simulink model "S600_stromregelung"  (Simulink 9.2)
settings: Solver=FixedStepDiscrete  StartTime=0.0  StopTime=inf  FixedStep=param.t_sample  RelTol=1e-3
undefined symbols (not defined in the file or in its folder): param
libraries: etherlab_lib x1
settings Model: Creator=schappler  LastModifiedBy=pkr_devpc  SimulationMode=external  ExtModeTrigDuration=10000  ExtModeArchiveMode=auto  ExtModeArchiveFileName=measurement_data  ExtModeArchiveDirName=/home/pkr_devpc/Schreibtisch/Git/3rrr_pkm/Versuchsstand/result  ExtModeLogAll=off
settings SolverCC: MinimalZcImpactIntegration=on
settings DataIOCC: LimitDataPoints=off  SaveFormat=Dataset  SignalLoggingSaveFormat=Dataset  SaveOutput=off  SignalLogging=off  SaveTime=off
settings OptimizationCC: BufferReuse=off  GlobalBufferReuse=off  ExpressionFolding=off  LocalBlockOutputs=off  LifeSpan=auto  OptimizeDataStoreBuffers=off  BusAssignmentInplaceUpdate=off
settings DebuggingCC: ReadBeforeWriteMsg=DisableAll  WriteAfterWriteMsg=DisableAll  WriteAfterReadMsg=DisableAll  UnderspecifiedInitializationDetection=Simplified  MergeDetectMultiDrivingBlocksExec=error  MultiTaskDSMMsg=none  FcnCallInpInsideContextMsg=error  StateNameClashWarn=none  SFUnexpectedBacktrackingDiag=error  SFNoUnconditionalDefaultTransitionDiag=error  SFExecutionAtInitializationDiag=warning
settings HardwareCC: ProdBitPerPointer=64  ProdBitPerSizeT=64  ProdBitPerPtrDiffT=64  ProdLargestAtomicFloat=Float  ProdIntDivRoundTo=Zero  ProdEndianess=LittleEndian  ProdWordSize=64  ProdHWDeviceType=Intel->x86-64 (Windows64)
settings ModelReferenceCC: UpdateModelReferenceTargets=IfOutOfDate  PropagateSignalLabelsOutOfModel=on
settings SFSimCC: SFSimEcho=off  SimUseLocalCustomCode=on
settings RTWCC: SystemTargetFile=etherlab.tlc  TemplateMakefile=etherlab_hrt.tmf  Description=EtherLab PREEMT_RT Real-Time Target  GenerateReport=on  RTWUseLocalCustomCode=on  LaunchReport=on
settings CodeAppCC: StateflowObjectComments=off
settings STFCustomTargetCC: TargetLangStandard=C99 (ISO)  SystemTargetFile=etherlab.tlc
settings GRTTargetCC: TargetLangStandard=C99 (ISO)  ParMdlRefBuildCompliant=off  CompOptLevelCompliant=off  ConcurrentExecutionCompliant=off  GeneratePreprocessorConditionals=Use local settings  MatFileLogging=off  CPPClassGenCompliant=off  UseToolchainInfoCompliant=off  ExtMode=on  ExtModeStaticAlloc=on  ExtModeStaticAllocSize=2000000000  ExtModeMexArgs='10.144.130.139' 0 17725  RTWCAPISignals=on  RTWCAPIParams=on
settings CustomProperty: DataType=int32  Value=2
settings ConfigComp: CovMetricSettings=dwe  CovHtmlReporting=off  CovSaveCumulativeToWorkspaceVar=off  CovSaveSingleToWorkspaceVar=off  CovExternalEMLEnable=on

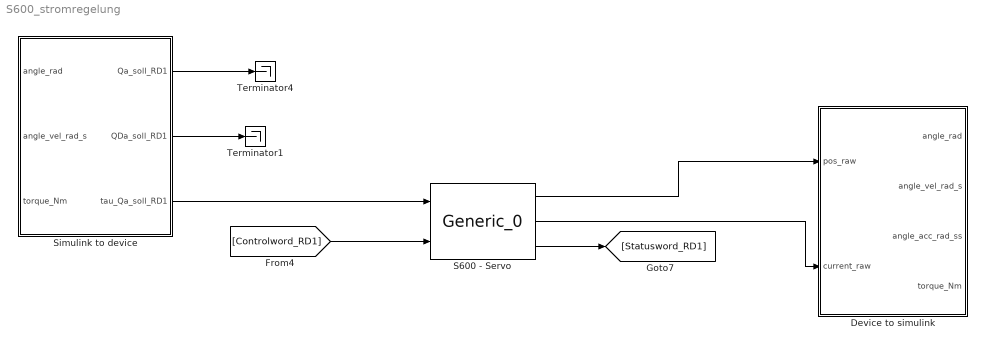
== system S600_stromregelung ==
  Device to simulink : Subsystem
  S600 - Servo : etherlab_lib/EtherCAT/Generic_0  master=0  index=1  rv=S600_stromregelung  param=[]  tsample=0.001  debug=0
  Simulink to device : Subsystem
  Terminator1 : Terminator
  Terminator4 : Terminator
  wires:
  S600 - Servo/1 -> Device to simulink/1(pos_raw)
  S600 - Servo/2 -> Device to simulink/2(current_raw)
  [Controlword_RD1] -> S600 - Servo/2
  S600 - Servo/3 -> [Statusword_RD1]
  Simulink to device/3(tau_Qa_soll_RD1) -> S600 - Servo/1
  Simulink to device/1(Qa_soll_RD1) -> Terminator4/1
  Simulink to device/2(QDa_soll_RD1) -> Terminator1/1

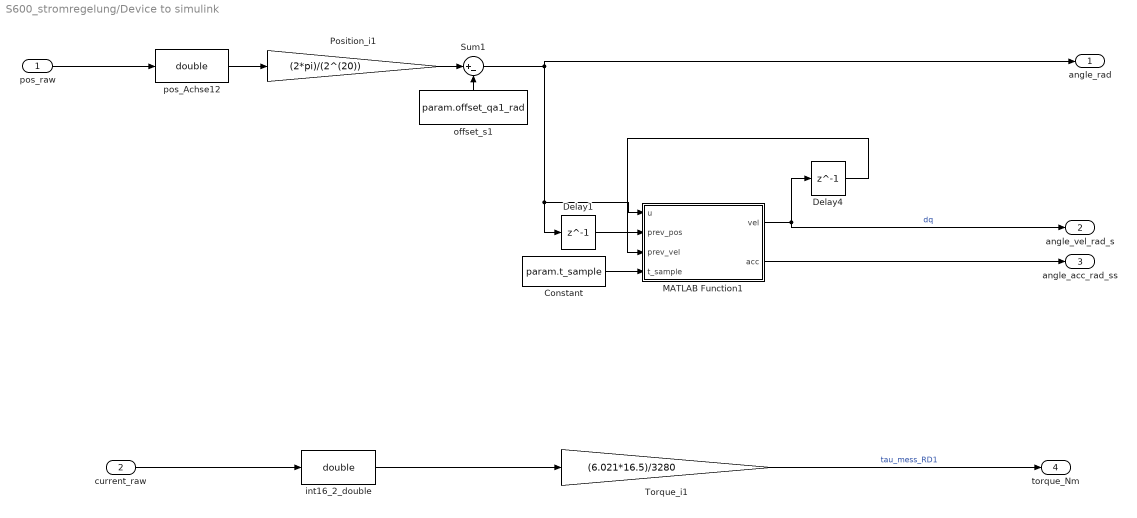
== system S600_stromregelung/Device to simulink ==
  pos_raw : Inport
  current_raw : Inport  Port=2
  Constant : Constant  Value=param.t_sample  SampleTime=-1
  Delay1 : Delay  DelayLength=1  InitialCondition=param.offset_qa1_rad
  Delay4 : Delay  DelayLength=1
  MATLAB Function1 : MATLAB Function  TreatAsAtomicUnit=on
  Position_i1 : Gain  Gain=(2*pi)/(2^(20))  ParamDataTypeStr=float('double')  OutDataTypeStr=float('double')
  Sum1 : Sum  Inputs=|+-
  Torque_i1 : Gain  Gain=(6.021*16.5)/3280  ParamDataTypeStr=float('double')  OutDataTypeStr=float('double')
  int16_2_double : DataTypeConversion  OutDataTypeStr=double
  offset_s1 : Constant  Value=param.offset_qa1_rad  SampleTime=-1
  pos_Achse12 : DataTypeConversion  OutDataTypeStr=double
  angle_rad : Outport  VectorParamsAs1DForOutWhenUnconnected=on
  angle_vel_rad_s : Outport  Port=2  VectorParamsAs1DForOutWhenUnconnected=on
  angle_acc_rad_ss : Outport  Port=3  VectorParamsAs1DForOutWhenUnconnected=on
  torque_Nm : Outport  Port=4  VectorParamsAs1DForOutWhenUnconnected=on
  wires:
  current_raw/1 -> int16_2_double/1
  Constant/1 -> MATLAB Function1/4(t_sample)
  Delay4/1 -> MATLAB Function1/3(prev_vel)
  pos_raw/1 -> pos_Achse12/1
  MATLAB Function1/1(vel) -> Delay4/1, angle_vel_rad_s/1  "dq"
  Delay1/1 -> MATLAB Function1/2(prev_pos)
  MATLAB Function1/2(acc) -> angle_acc_rad_ss/1
  Torque_i1/1 -> torque_Nm/1  "tau_mess_RD1"
  pos_Achse12/1 -> Position_i1/1
  offset_s1/1 -> Sum1/2
  Position_i1/1 -> Sum1/1
  Sum1/1 -> angle_rad/1, Delay1/1, MATLAB Function1/1(u)
  int16_2_double/1 -> Torque_i1/1

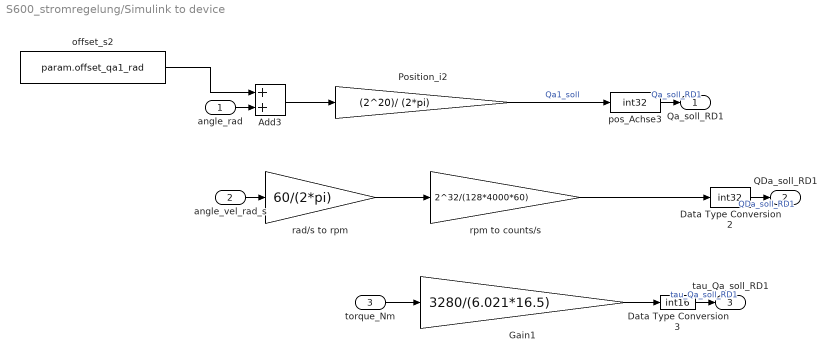
== system S600_stromregelung/Simulink to device ==
  angle_rad : Inport
  angle_vel_rad_s : Inport  Port=2
  torque_Nm : Inport  Port=3
  Add3 : Sum
  Data Type Conversion2 : DataTypeConversion  OutDataTypeStr=int32
  Data Type Conversion3 : DataTypeConversion  OutDataTypeStr=int16
  Gain1 : Gain  Gain=3280/(6.021*16.5)
  Position_i2 : Gain  Gain=(2^20)/ (2*pi)  ParamDataTypeStr=float('double')  OutDataTypeStr=float('double')
  offset_s2 : Constant  Value=param.offset_qa1_rad  SampleTime=-1
  pos_Achse3 : DataTypeConversion  OutDataTypeStr=int32
  rad/s to rpm : Gain  Gain=60/(2*pi)
  rpm to counts/s : Gain  Gain=2^32/(128*4000*60)
  Qa_soll_RD1 : Outport
  QDa_soll_RD1 : Outport  Port=2
  tau_Qa_soll_RD1 : Outport  Port=3
  wires:
  angle_rad/1 -> Add3/2
  Gain1/1 -> Data Type Conversion3/1
  pos_Achse3/1 -> Qa_soll_RD1/1  "Qa_soll_RD1"
  rpm to counts/s/1 -> Data Type Conversion2/1
  angle_vel_rad_s/1 -> rad/s to rpm/1
  Data Type Conversion2/1 -> QDa_soll_RD1/1  "QDa_soll_RD1"
  Data Type Conversion3/1 -> tau_Qa_soll_RD1/1  "tau_Qa_soll_RD1"
  offset_s2/1 -> Add3/1
  Add3/1 -> Position_i2/1
  Position_i2/1 -> pos_Achse3/1  "Qa1_soll"
  torque_Nm/1 -> Gain1/1
  rad/s to rpm/1 -> rpm to counts/s/1

== matlab function Device to simulink/MATLAB Function1 ==
  data: u input double; vel output double; prev_pos input double; prev_vel input double; t_sample input double; acc output double
function [vel, acc] = fcn(u, prev_pos, prev_vel, t_sample)

vel = (u-prev_pos)/t_sample;
acc = (vel-prev_vel)/t_sample;
